simulink model "asgm2_exc1"  (R2024a)
settings: Solver=VariableStepAuto  StartTime=0.0  StopTime=20  RelTol=1e-3
undefined symbols (not defined in the file): A, B, C, Ex, Fx, Fy, WTfq, X0
settings Model: Creator=HIEDA  LastModifiedBy=HIEDA

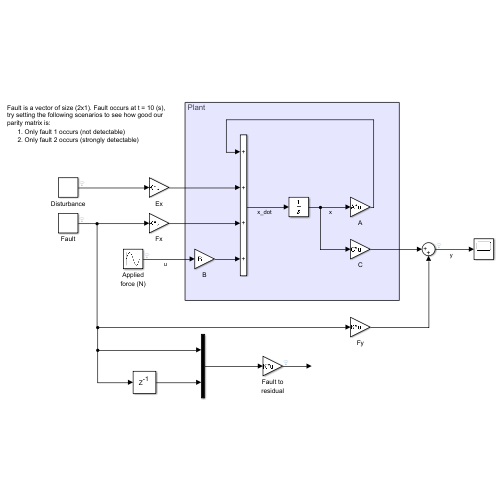
[thumbnail: Simulink's stored preview of the top-level diagram]
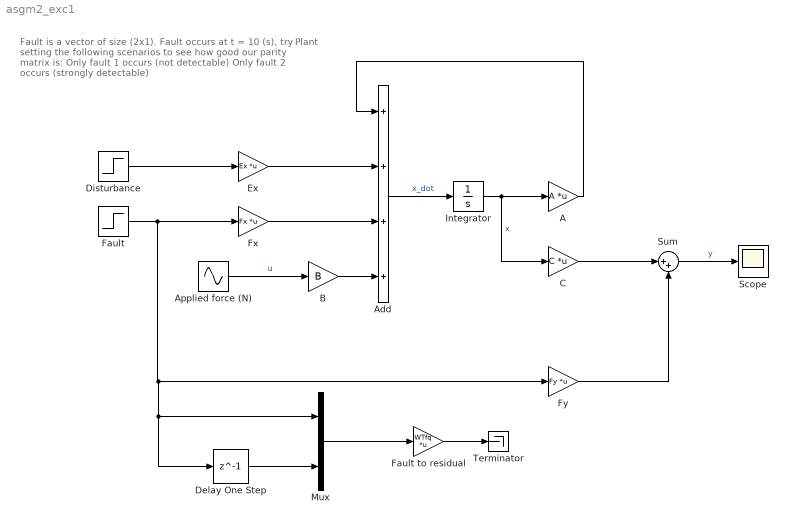
== system asgm2_exc1 ==
  note: Fault is a vector of size (2x1). Fault occurs at t = 10 (s), try setting the following scenarios to see how good our parity matrix is:
      | Only fault 1 occurs (not detectable)
      | Only fault 2 occurs (strongly detectable)
  note: Plant
  A : Gain  Gain=A  Multiplication=Matrix(K*u)
  Add : Sum  Inputs=++++
  Applied force (N) : Sin  Amplitude=2  Frequency=0.5  SampleTime=0
  B : Gain  Gain=B
  C : Gain  Gain=C  Multiplication=Matrix(K*u)
  Delay One Step : Delay  DelayLength=1
  Disturbance : Step  Time=10  After=0.12  SampleTime=0
  Ex : Gain  Gain=Ex  Multiplication=Matrix(K*u)
  Fault : Step  Time=10  Before=[0; 0]  After=[0; 0.5]  SampleTime=0
  Fault to residual : Gain  Gain=WTfq  Multiplication=Matrix(K*u)
  Fx : Gain  Gain=Fx  Multiplication=Matrix(K*u)
  Fy : Gain  Gain=Fy  Multiplication=Matrix(K*u)
  Integrator : Integrator  InitialCondition=X0
  Mux : Mux  Inputs=2
  Scope : Scope
  Sum : Sum  Inputs=|++
  Terminator : Terminator
  wires:
  B/1 -> Add/4
  Add/1 -> Integrator/1  "x_dot"
  Integrator/1 -> A/1, C/1  "x"
  A/1 -> Add/1
  Disturbance/1 -> Ex/1
  Ex/1 -> Add/2
  Fault/1 -> Delay One Step/1, Mux/1, Fy/1, Fx/1
  Fx/1 -> Add/3
  C/1 -> Sum/1
  Fy/1 -> Sum/2
  Sum/1 -> Scope/1  "y"
  Fault to residual/1 -> Terminator/1
  Applied force (N)/1 -> B/1  "u"
  Mux/1 -> Fault to residual/1
  Delay One Step/1 -> Mux/2
